simulink model "application_3"  (R2017b)
settings: Solver=VariableStepAuto  StartTime=0.0  StopTime=16  RelTol=1e-3
libraries: simulink_extras x4
settings Model: Creator=exybore  LastModifiedBy=exybore

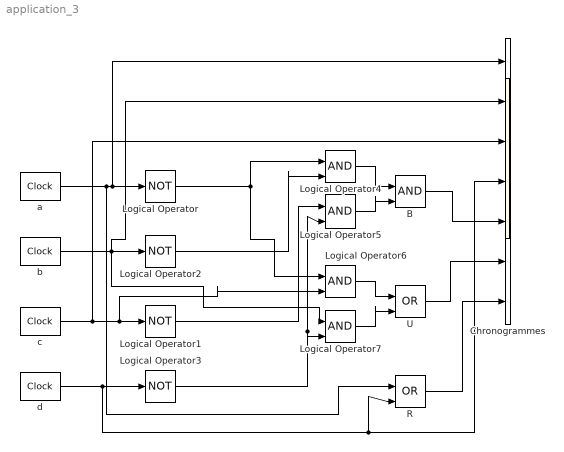
== system application_3 ==
  B : Logic  IconShape=distinctive  AllPortsSameDT=off  OutDataTypeStr=boolean
  Chronogrammes : Scope  NumInputPorts=7
  Logical Operator{,1..3} (4 alike) : Logic  Operator=NOT  IconShape=distinctive  AllPortsSameDT=off  OutDataTypeStr=boolean
  Logical Operator{4..7} (4 alike) : Logic  IconShape=distinctive  AllPortsSameDT=off  OutDataTypeStr=boolean
  R : Logic  Operator=OR  IconShape=distinctive  AllPortsSameDT=off  OutDataTypeStr=boolean
  U : Logic  Operator=OR  IconShape=distinctive  AllPortsSameDT=off  OutDataTypeStr=boolean
  a : simulink_extras/Flip Flops/Clock  period=16
  b : simulink_extras/Flip Flops/Clock  period=8
  c : simulink_extras/Flip Flops/Clock  period=4
  d : simulink_extras/Flip Flops/Clock  period=2
  wires:
  b/1 -> Logical Operator7/1, Chronogrammes/2, Logical Operator2/1
  a/1 -> Chronogrammes/1, Logical Operator/1, R/1
  c/1 -> Chronogrammes/3, Logical Operator6/2, Logical Operator1/1
  d/1 -> R/2, Chronogrammes/4, Logical Operator3/1
  Logical Operator/1 -> Logical Operator4/1, Logical Operator6/1
  Logical Operator2/1 -> Logical Operator4/2
  Logical Operator1/1 -> Logical Operator5/1
  Logical Operator3/1 -> Logical Operator5/2, Logical Operator7/2
  Logical Operator4/1 -> B/1
  Logical Operator5/1 -> B/2
  B/1 -> Chronogrammes/5
  U/1 -> Chronogrammes/6
  Logical Operator6/1 -> U/1
  Logical Operator7/1 -> U/2
  R/1 -> Chronogrammes/7
